simulink model "ConnectionUsingBytes"  (R2025b)
settings: Solver=FixedStepAuto  StartTime=0.0  StopTime=inf  FixedStep=0.01  RelTol=1e-3
undefined symbols (not defined in the file or in its folder): LF
libraries: instrumentseriallib x4, etargetslib x2, simulink x1
settings Model: Creator=talles  LastModifiedBy=a_jax

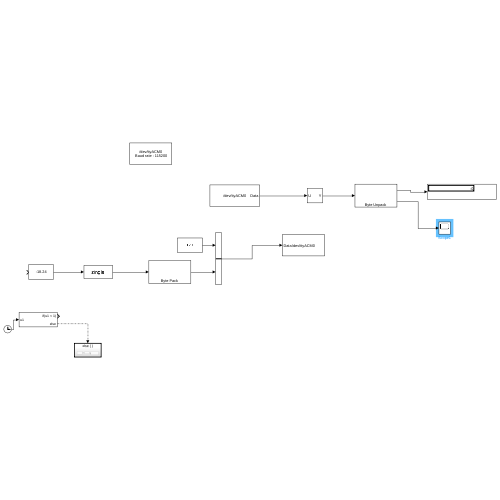
[thumbnail: Simulink's stored preview of the top-level diagram]
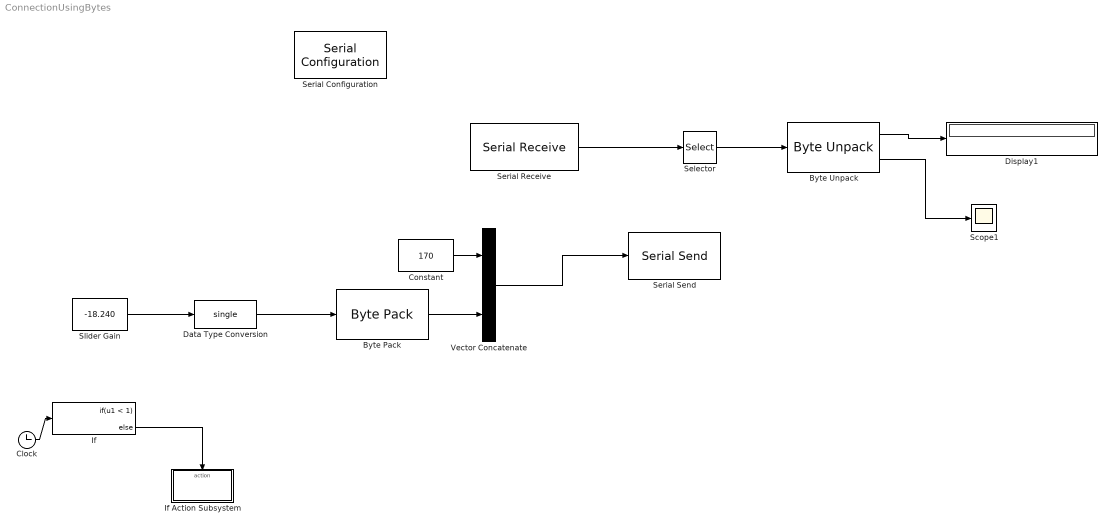
== system ConnectionUsingBytes ==
  Byte Pack : etargetslib/Byte Pack  datatypes={'single'}  byteAlign=4
  Byte Unpack : etargetslib/Byte Unpack  dimensions={1, 1}  datatypes={'single', 'int32'}  byteAlign=4
      settings: LibrarySourceBlock=embeddedtargetslib/Host Communication/Byte Unpack
  Clock : Clock
  Constant : Constant  Value=170  OutDataTypeStr=uint8
  Data Type Conversion : DataTypeConversion  OutDataTypeStr=single  SaturateOnIntegerOverflow=off  RndMeth=Floor
  Display1 : Display
  If : If  IfExpression=u1 < 1
  If Action Subsystem : Subsystem  TreatAsAtomicUnit=on
  Scope1 : Scope
      settings: ActiveDisplayYMinimum=-1.9345327032385473E+9  ActiveDisplayYMaximum=1.4635628972057686E+9
  Selector : Selector  InputPortWidth=9  IndexOptions=Index vector (dialog)  Indices=2:9  OutputSizes=1
  Serial Configuration : instrumentseriallib/Serial Configuration  Priority=-200000  PortSel=/dev/ttyACM0  Port=/dev/ttyACM0  ComPort=/dev/ttyACM0  BaudRate=115200  DataBits=8  Parity=none  StopBits=1  ByteOrder=little-endian  FlowControl=none  Timeout=0.0001  SimulateUsing=Interpreted execution  BlockInModel=on  aMode=1
      settings: LibrarySourceBlock=embeddedtargetslib/Host Communication/Serial Configuration
  Serial Receive : instrumentseriallib/Serial Receive  Priority=1  PortSel=/dev/ttyACM0  Port=/dev/ttyACM0  ComPort=/dev/ttyACM0  DataType=uint8  SaveDataType=uint8  ToggleHeader=off  Header=[10]  ToggleDataSize=on  DataSize=[9]  ToggleTerminator=off  Terminator=LF ('\n')  CustomTerminator=[]  InputFormat=Column major  EnableBlockingMode=on  ActionDataUnavailable=Output last received value  ActionWhenDataUnavailable=Output last received value  CustomValue=0  SampleTime=0.01  SimulateUsing=Interpreted execution  BlockInModel=on  aMode=1  LibraryInUse=instrumentlib
  Serial Send : instrumentseriallib/Serial Send  Priority=1  PortSel=/dev/ttyACM0  Port=/dev/ttyACM0  ComPort=/dev/ttyACM0  Header=[]  Terminator=LF ('\n')  CustomTerminator=[]  EnableBlockingMode=on  SimulateUsing=Interpreted execution  BlockInModel=on  aMode=1
      settings: LibrarySourceBlock=embeddedtargetslib/Host Communication/Serial Send
  Slider Gain : simulink/Math Operations/Slider Gain  gain=-18.240  low=-24  high=24
  Vector Concatenate : Concatenate
  wires:
  Serial Receive/1 -> Selector/1
  Clock/1 -> If/1
  If/2 -> If Action Subsystem/Action
  Slider Gain/1 -> Data Type Conversion/1
  Data Type Conversion/1 -> Byte Pack/1
  Constant/1 -> Vector Concatenate/1
  Byte Pack/1 -> Vector Concatenate/2
  Vector Concatenate/1 -> Serial Send/1
  Selector/1 -> Byte Unpack/1
  Byte Unpack/1 -> Display1/1
  Byte Unpack/2 -> Scope1/1

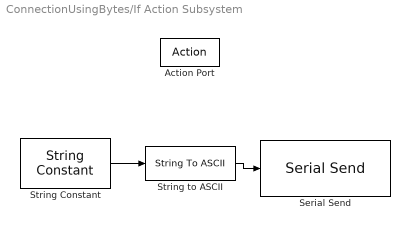
== system ConnectionUsingBytes/If Action Subsystem ==
  Action Port : ActionPort  ActionPortLabel=else
  Serial Send : instrumentseriallib/Serial Send  Priority=1  PortSel=/dev/ttyACM0  Port=/dev/ttyACM0  ComPort=/dev/ttyACM0  Header=[]  Terminator=LF ('\n')  CustomTerminator=[]  EnableBlockingMode=on  SimulateUsing=Interpreted execution  BlockInModel=on  aMode=1
  String Constant : StringConstant  String="\"1111,5556\""
  String to ASCII : StringToASCII
  wires:
  String Constant/1 -> String to ASCII/1
  String to ASCII/1 -> Serial Send/1
